simulink model "loopShaping"  (Simulink 8.8)
settings: Solver=ode45  StartTime=0.0  StopTime=10  RelTol=1e-3  EnableMultiTasking=on
values from neighbouring files (symbols this model uses):
  A = [0 1; 0 -c/m]    [Untitled2.m]    (also in define_consts.m; loadProperties.m; t.mat = [0  1; 0  -0.025]; test.m)
  a = 0.1    [LoopShapingFilter.m]    (also in LoopShapingFilterNoisy.m; LoopShapingLeadCompensator.m = as(i); LoopShapingPIController.m; Untitled2.m)
  B = [0;1/m]    [Untitled2.m]    (also in define_consts.m; loadProperties.m; t.mat = [0 0.1]; test.m = [0 0;1/m 0])
  C = [1 0]    [Untitled2.m]    (also in deadline4.m = tf([4, 1],[0, 2]); define_consts.m; loadProperties.m; t.mat)
  G0 = getGain(Hcontroller * P, wco)    [LoopShapingFilter.m]    (also in LoopShapingFilterNoisy.m; LoopShapingFinal.m = getGain(P, wco); LoopShapingLeadCompensator.m = getGain(H, wco); LoopShapingPIController.m)
  s = ss(A,B,C,D)    [LoopShapingFinal.m]    (also in LoopShapingFinalCrossover.m; LoopShapingNoise.m; LoopShapingTest.m; LoopsShapingCrossover.m)
  wco = 5    [LoopShapingFilter.m]    (also in LoopShapingFilterNoisy.m = 3; LoopShapingFinal.m = 7.2; LoopShapingLeadCompensator.m = 7.24; LoopShapingPIController.m = 3)
libraries: commchan3 x2, slctrlblks x1
settings Model: LogicAnalyzerSignalOrdering=90daa040-f722-4977-9d6a-0050db127c74,8d65b11b-61c5-4494-877e-e1d3003be209,42e16e0e-1eea-4d86-bca9-c5718df0c75f,563aebda-9530-45ab-9ae4-6dceb17a15c5  Creator=Adrien  LastModifiedBy=Adrien
settings DataIOCC: SignalLoggingSaveFormat=Dataset
settings DebuggingCC: UnderspecifiedInitializationDetection=Simplified  MergeDetectMultiDrivingBlocksExec=error  FcnCallInpInsideContextMsg=error  StateNameClashWarn=none
settings GRTTargetCC: CombineOutputUpdateFcns=on  GRTInterface=off

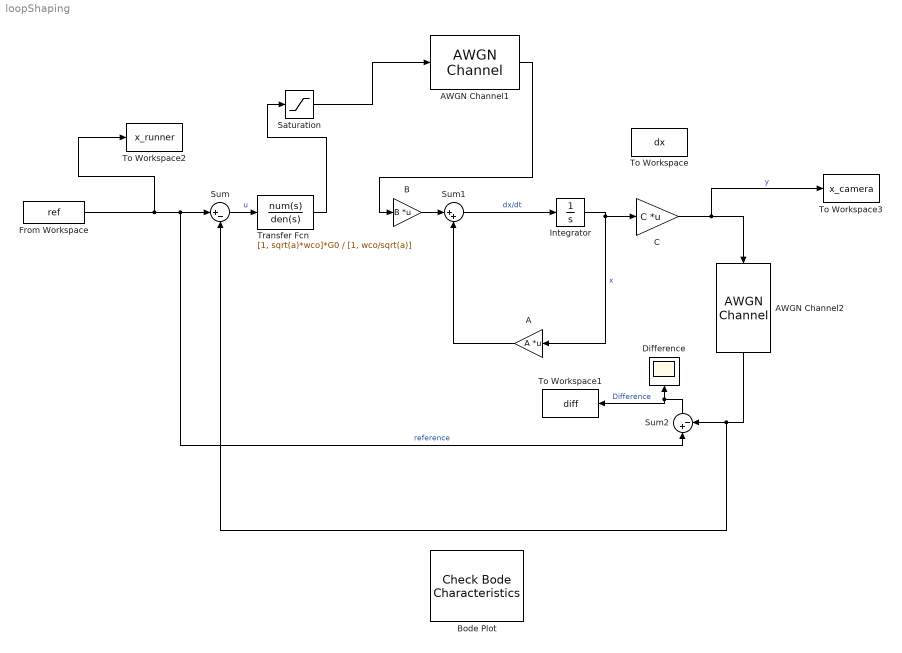
== system loopShaping ==
  A : Gain  Gain=A  Multiplication=Matrix(K*u)
  AWGN Channel1 : commchan3/AWGN Channel  InputProcessing=Columns as channels (frame based)  seed=67  noiseMode=Variance from mask  EbNodB=10  EsNodB=10  SNRdB=10  bitsPerSym=1  Ps=1  Tsym=1  variance=d
  AWGN Channel2 : commchan3/AWGN Channel  InputProcessing=Columns as channels (frame based)  seed=67  noiseMode=Variance from mask  EbNodB=10  EsNodB=10  SNRdB=10  bitsPerSym=1  Ps=1  Tsym=1  variance=n
  "B  " : Gain  Gain=B  Multiplication=Matrix(K*u)
  Bode Plot : slctrlblks/Model Verification/Check Bode  Characteristics  InstantiateOnLoad=on  SaveOperatingPoints=off  LinearizationIOs={'/Sum', 1, 'in', 'off', '';'/C ', 1, 'out', 'on', ''}  LinearizeAt=SnapshotTimes  SnapshotTimes=[0]  TriggerType=rising  SampleTime=auto  RateConversionMethod=zoh  PreWarpFreq=10  UseExactDelayModel=off  UseFullBlockNameLabels=off  UseBusSignalLabels=off  enabled=on  stopWhenAssertionFail=off  export=off  ViewDlgPos=[]  OpenViewOnLoad=off  LaunchViewOnOpen=off  FrequencyUnits=rad/s  MagnitudeUnits=dB  PhaseUnits=deg  TimeUnits=seconds  EnableUpperBound=off  UpperBoundFrequencies=[]  UpperBoundMagnitudes=[]  EnableLowerBound=off  LowerBoundFrequencies=[]  LowerBoundMagnitudes=[]
      settings: SaveToWorkspace=on
  "C " : Gain  Gain=C  Multiplication=Matrix(K*u)
  Difference : Scope
  From Workspace : FromWorkspace  VariableName=ref  SampleTime=step  Interpolate=off  OutputAfterFinalValue=Holding final value
  Integrator : Integrator  InitialCondition=[0 0]
  Saturation : Saturate  UpperLimit=70  LowerLimit=-70
  Sum : Sum  Inputs=|+-
  Sum1 : Sum  Inputs=|++
  Sum2 : Sum  Inputs=|+-
  To Workspace : ToWorkspace  VariableName=dx  SaveFormat=Timeseries  SampleTime=-1
  To Workspace1 : ToWorkspace  VariableName=diff  SaveFormat=Timeseries  SampleTime=-1
  To Workspace2 : ToWorkspace  VariableName=x_runner  SaveFormat=Timeseries  SampleTime=-1
  To Workspace3 : ToWorkspace  VariableName=x_camera  SaveFormat=Timeseries  SampleTime=-1
  Transfer Fcn : TransferFcn  Numerator=[1, sqrt(a)*wco]*G0  Denominator=[1, wco/sqrt(a)]
  wires:
  Integrator/1 -> A/1, "C "/1  "x"
  "B  "/1 -> Sum1/1
  A/1 -> Sum1/2
  From Workspace/1 -> Sum/1, Sum2/1, To Workspace2/1  "reference"
  "C "/1 -> To Workspace3/1, AWGN Channel2/1  "y"
  Sum1/1 -> Integrator/1  "dx/dt"
  Sum2/1 -> To Workspace1/1, Difference/1  "Difference"
  Sum/1 -> Transfer Fcn/1  "u"
  Transfer Fcn/1 -> Saturation/1
  Saturation/1 -> AWGN Channel1/1
  AWGN Channel1/1 -> "B  "/1
  AWGN Channel2/1 -> Sum2/2, Sum/2
